simulink model "testFrame_PWMtoAngle"  (R2020b)
settings: Solver=FixedStepDiscrete  StartTime=0.0  StopTime=2  FixedStep=200e-6  RelTol=1e-3
libraries: simulink x2, simulink_extras x1
settings Model: SnapshotBufferSize=50  SnapshotInterval=1  Creator=unix  LastModifiedBy=unix
settings DebuggingCC: IntegerOverflowMsg=error  ParameterUnderflowMsg=error  IntegerSaturationMsg=error

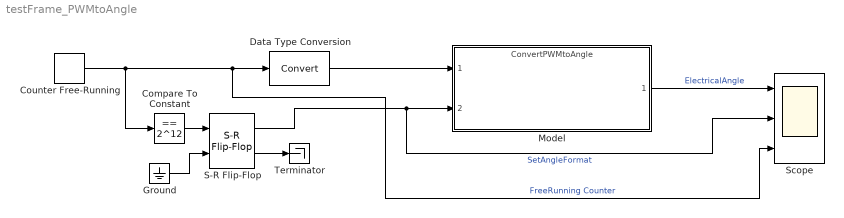
== system testFrame_PWMtoAngle ==
  Compare To Constant : simulink/Logic and Bit Operations/Compare To Constant  relop===  const=2^12  OutDataTypeStr=boolean
  Counter Free-Running : simulink/Sources/Counter Free-Running  NumBits=12  tsamp=-1
  Data Type Conversion : DataTypeConversion
  Ground : Ground
  Model : ModelReference  ModelNameDialog=ConvertPWMtoAngle.slx  ModelReferenceVersion=3.4
  S-R Flip-Flop : simulink_extras/Flip Flops/S-R Flip-Flop  initial_condition=0
  Scope : Scope  NumInputPorts=3
  Terminator : Terminator
  wires:
  Counter Free-Running/1 -> Scope/3, Data Type Conversion/1, Compare To Constant/1  "FreeRunning Counter"
  Data Type Conversion/1 -> Model/1
  Model/1 -> Scope/1  "ElectricalAngle"
  S-R Flip-Flop/1 -> Scope/2, Model/2  "SetAngleFormat"
  S-R Flip-Flop/2 -> Terminator/1
  Compare To Constant/1 -> S-R Flip-Flop/1
  Ground/1 -> S-R Flip-Flop/2
